simulink model "function_teste22"  (Simulink 8.0)
settings: Solver=ode45  StartTime=0.0  StopTime=20.0  FixedStep=20.0/100  RelTol=1e-9
values from neighbouring files (symbols this model uses):
  alpha1 = x_c(2)    [Lab1.m]
  alpha2 = 1.2    [Lab1.m]
  delta1 = -1.2    [Lab1.m]
  delta2 = 2.3    [Lab1.m]
  N1_0 = x_c(1)    [Lab1.m]
  N2_0 = 10    [Lab1.m]
settings Model: Creator=Katarina  LastModifiedBy=Katarina
settings DataIOCC: LimitDataPoints=off  MaxDataPoints=101
settings DebuggingCC: SolverPrmCheckMsg=none

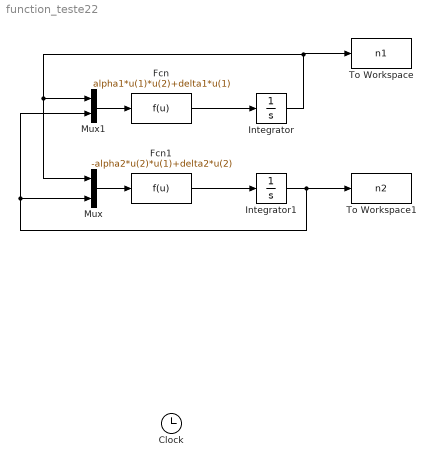
== system function_teste22 ==
  Fcn : Fcn  Expr=alpha1*u(1)*u(2)+delta1*u(1)
  Fcn1 : Fcn  Expr=-alpha2*u(2)*u(1)+delta2*u(2)
  Integrator : Integrator  InitialCondition=N1_0
  Integrator1 : Integrator  InitialCondition=N2_0
  Mux : Mux  Inputs=2
  Mux1 : Mux  Inputs=2
  To Workspace : ToWorkspace  VariableName=n1  SampleTime=-1
  To Workspace1 : ToWorkspace  VariableName=n2  SampleTime=-1
  Clock : Clock
      settings: IOType=siggen
  wires:
  Mux1/1 -> Fcn/1
  Mux/1 -> Fcn1/1
  Fcn/1 -> Integrator/1
  Integrator/1 -> Mux/1, Mux1/1, To Workspace/1
  Fcn1/1 -> Integrator1/1
  Integrator1/1 -> Mux/2, Mux1/2, To Workspace1/1
